simulink model "fuzzy_pid_simulink"  (R2020a)
settings: Solver=ode23tb  StartTime=0.0  StopTime=100  RelTol=1e-3  EnableMultiTasking=on
values from neighbouring files (symbols this model uses):
  fuzzy_K0 = Kp / Ti    (= 0.155906883029)    [fuzzy_pid.m]
  fuzzy_K1 = fuzzy_K0 * alpha_beta(2)    [fuzzy_pid.m]
  fuzzy_Kd = alpha_beta(2) * fuzzy_Ke    [fuzzy_pid.m]
  fuzzy_Ke = 1    [fuzzy_pid.m]
  Kp = 0.6 * Kcr    (= 0.545674090601)    [fuzzy_pid.m]
  Tcr = 7    [fuzzy_pid.m]
  Td = Tcr / 8    (= 0.875)    [fuzzy_pid.m]
  Ti = Tcr / 2    (= 3.5)    [fuzzy_pid.m]
libraries: fuzblock x1
settings Model: Creator=paulo.costa  LastModifiedBy=paulo
settings DataIOCC: LimitDataPoints=on  SaveFormat=Array  ReturnWorkspaceOutputs=off
settings OptimizationCC: LifeSpan=inf
settings DebuggingCC: UnderspecifiedInitializationDetection=Classic  MergeDetectMultiDrivingBlocksExec=none  SolverPrmCheckMsg=warning  StateNameClashWarn=warning  SFUnexpectedBacktrackingDiag=warning  SFNoUnconditionalDefaultTransitionDiag=warning  SFExecutionAtInitializationDiag=none  ArithmeticOperatorsInVariantConditions=warning
settings HardwareCC: ProdBitPerPointer=32  ProdBitPerSizeT=32  ProdBitPerPtrDiffT=32  ProdLargestAtomicFloat=None  ProdIntDivRoundTo=Undefined  ProdEndianess=Unspecified  ProdWordSize=32  ProdHWDeviceType=32-bit Generic
settings ModelReferenceCC: PropagateSignalLabelsOutOfModel=off
settings SFSimCC: SimUseLocalCustomCode=off  CustomCodeUndefinedFunction=UseInterfaceOnly
settings RTWCC: RTWUseLocalCustomCode=off
settings CodeAppCC: StateflowObjectComments=on
settings GRTTargetCC: TargetLangStandard=C89/C90 (ANSI)
settings ConfigComp: CovMetricSettings=dw  CovHtmlReporting=on  CovSaveCumulativeToWorkspaceVar=on  CovSaveSingleToWorkspaceVar=on  CovExternalEMLEnable=off

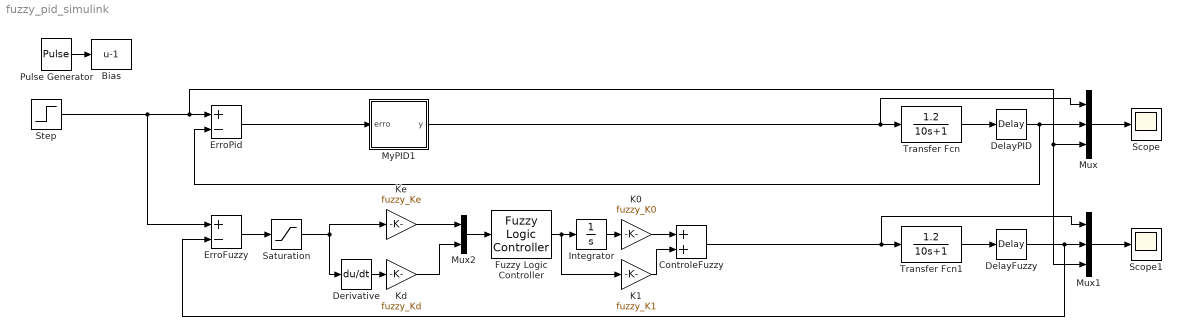
== system fuzzy_pid_simulink ==
  Bias : Bias  Bias=-1
  ControleFuzzy : Sum
  DelayFuzzy : TransportDelay  DelayTime=2
  DelayPID : TransportDelay  DelayTime=2
  Derivative : Derivative
  ErroFuzzy : Sum  Inputs=+-
  ErroPid : Sum  Inputs=+-
  Fuzzy Logic Controller : fuzblock/Fuzzy Logic  Controller  FIS=fuzzy_pid  OutputSampleNumber=101  DataType=double  FuzzifiedInputs=off  RuleFiringStrengths=off  RuleOutputs=off  AggregatedOutputs=off  SimulateUsing=Interpreted execution  OutOfRangeInputValueMessage=warning  NoRuleFiredMessage=warning  EmptyOutputFuzzySetMessage=warning
  Integrator : Integrator
  K0 : Gain  Gain=fuzzy_K0
  K1 : Gain  Gain=fuzzy_K1
  Kd : Gain  Gain=fuzzy_Kd
  Ke : Gain  Gain=fuzzy_Ke
  Mux : Mux  Inputs=3
  Mux1 : Mux  Inputs=3
  Mux2 : Mux  Inputs=2
  MyPID1 : Subsystem
  Pulse Generator : DiscretePulseGenerator  PulseType=Time based  Amplitude=2  Period=Tcr  PulseWidth=50
  Saturation : Saturate  UpperLimit=1  LowerLimit=-1
  Scope : Scope
  Scope1 : Scope
  Step : Step  SampleTime=0
  Transfer Fcn : TransferFcn  Numerator=[1.2]  Denominator=[10 1]
  Transfer Fcn1 : TransferFcn  Numerator=[1.2]  Denominator=[10 1]
  wires:
  Mux/1 -> Scope/1
  DelayFuzzy/1 -> ErroFuzzy/2, Mux1/2
  Mux1/1 -> Scope1/1
  Fuzzy Logic Controller/1 -> K1/1, Integrator/1
  ErroFuzzy/1 -> Saturation/1
  Mux2/1 -> Fuzzy Logic Controller/1
  DelayPID/1 -> ErroPid/2, Mux/2
  ErroPid/1 -> MyPID1/1(erro)
  Step/1 -> Mux/3, Mux1/3, ErroPid/1, ErroFuzzy/1
  MyPID1/1(y) -> Mux/1, Transfer Fcn/1
  K0/1 -> ControleFuzzy/1
  K1/1 -> ControleFuzzy/2
  ControleFuzzy/1 -> Transfer Fcn1/1, Mux1/1
  Integrator/1 -> K0/1
  Ke/1 -> Mux2/1
  Transfer Fcn/1 -> DelayPID/1
  Transfer Fcn1/1 -> DelayFuzzy/1
  Derivative/1 -> Kd/1
  Kd/1 -> Mux2/2
  Saturation/1 -> Derivative/1, Ke/1
  Pulse Generator/1 -> Bias/1

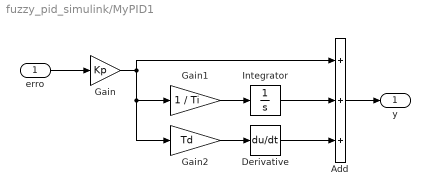
== system fuzzy_pid_simulink/MyPID1 ==
  erro : Inport
  Add : Sum  Inputs=+++
  Derivative : Derivative
  Gain : Gain  Gain=Kp
  Gain1 : Gain  Gain=1 / Ti
  Gain2 : Gain  Gain=Td
  Integrator : Integrator
  y : Outport
  wires:
  erro/1 -> Gain/1
  Gain/1 -> Gain2/1, Gain1/1, Add/1
  Gain1/1 -> Integrator/1
  Integrator/1 -> Add/2
  Gain2/1 -> Derivative/1
  Derivative/1 -> Add/3
  Add/1 -> y/1
